simulink model "ASW_PhVltgGen"  (R2023a)
settings: configuration reference "cfg_FastTaskCodeGeneration_v01" (kept outside this file)
undefined symbols (not defined in the file): Cdbl_tiMedTaskSmpTi
settings Model: DataDictionary=dd_foc_dictionary.sldd  EnableAccessToBaseWorkspace=off  Creator=WFYXQ  LastModifiedBy=xiaoqiang.yuan
settings ConfigSetRef: SourceName=cfg_FastTaskCodeGeneration_v01

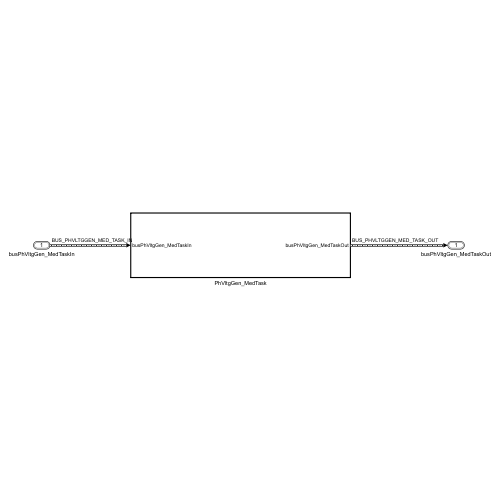
[thumbnail: Simulink's stored preview of the top-level diagram]
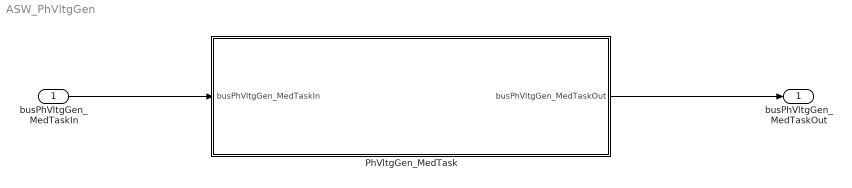
== system ASW_PhVltgGen ==
  busPhVltgGen_MedTaskIn : Inport  OutDataTypeStr=Bus: BUS_PHVLTGGEN_MED_TASK_IN  SampleTime=round(double(Cdbl_tiMedTaskSmpTi),6)  BusOutputAsStruct=on
  PhVltgGen_MedTask : Subsystem  TreatAsAtomicUnit=on  RTWFcnName=PhVltgGen_MedTask
      settings: RTWSystemCode=Nonreusable function  RTWFcnNameOpts=User specified
  busPhVltgGen_MedTaskOut : Outport  OutDataTypeStr=Bus: BUS_PHVLTGGEN_MED_TASK_OUT  SampleTime=round(double(Cdbl_tiMedTaskSmpTi),6)
  wires:
  busPhVltgGen_MedTaskIn/1 -> PhVltgGen_MedTask/1(busPhVltgGen_MedTaskIn)
  PhVltgGen_MedTask/1(busPhVltgGen_MedTaskOut) -> busPhVltgGen_MedTaskOut/1

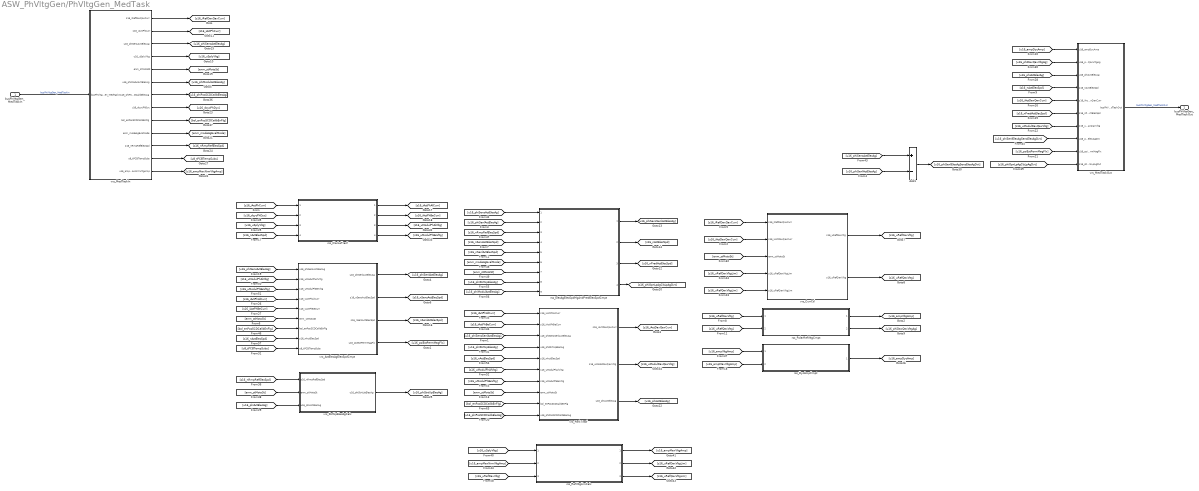
== system ASW_PhVltgGen/PhVltgGen_MedTask ==
  busPhVltgGen_MedTaskIn : Inport
  Add1 : Sum  InitFcn=|  Inputs=+-  OutDataTypeStr=Inherit: Same as first input
      | Simulink.suppressDiagnostic(gcb,...
      | 'SimulinkFixedPoint:util:Overflowoccurred');
  rss_ClarkeTrasf : Subsystem  ReferencedSubsystem=rss_ClarkeTrasf
  rss_DycAmpCmpt : Subsystem  ReferencedSubsystem=rss_DycAmpCmpt
  rss_ElecAgElecSpdMgAndPredElecSpdCmpt : Subsystem  VariantControl=Choice  ReferencedSubsystem=rss_ElecAgElecSpdMgAndPredElecSpdCmpt
  rss_PolarRefVltgCmpt : Subsystem  ReferencedSubsystem=rss_PolarRefVltgCmpt
  rss_RefVltgLimCalc : Subsystem  ReferencedSubsystem=rss_RefVltgLimCalc
  vrs_ActElecAgElecSpdCmpt : Subsystem  Variant=on  VariantControlMode=label  VariantControl=Choice  LabelModeActiveChoice=cstHybrCtrlLbl
  vrs_CurrCtl : Subsystem  Variant=on  VariantControlMode=label  VariantControl=Choice  LabelModeActiveChoice=cstSensCtrlLbl
  vrs_MedTaskIn : Subsystem  Variant=on  VariantControlMode=label  VariantControl=Choice  LabelModeActiveChoice=cstHybrCtrlLbl
  vrs_MedTaskOut : Subsystem  Variant=on  VariantControlMode=label  VariantControl=Choice  LabelModeActiveChoice=cstHybrCtrlLbl
  vrs_ParkTrasf : Subsystem  Variant=on  VariantControlMode=label  VariantControl=cstSensCtrlLbl  LabelModeActiveChoice=cstHybrCtrlLbl
  vrs_StrtUpElecAgCalc : Subsystem  Variant=on  VariantControlMode=label  LabelModeActiveChoice=cstSenlCtrlLbl
  busPhVltgGen_MedTaskOut : Outport
  wires:
  [s16_uModulPhBeVltg] -> vrs_ActElecAgElecSpdCmpt/3(s16_uModulPhBeVltg)
  vrs_MedTaskIn/1(s16_iRefDaxQaxCurr) -> [s16_iRefDaxQaxCurr]
  vrs_MedTaskOut/1(busPhVltgGen_MedTaskOut) -> busPhVltgGen_MedTaskOut/1  "busPhVltgGen_MedTaskOut"
  [u16_phiSensActElecAg] -> vrs_ActElecAgElecSpdCmpt/1(u16_phiSensActElecAg)
  [s16_iActPhCurr] -> rss_ClarkeTrasf/1
  vrs_MedTaskIn/4(u16_uSplyVltg) -> [u16_uSplyVltg]
  [s16_iActDaxQaxCurr] -> vrs_CurrCtl/2(s16_iActDaxQaxCurr)
  [u16_uSplyVltg] -> rss_ClarkeTrasf/3
  vrs_CurrCtl/2(s16_uRefQaxVltg) -> [s16_uRefQaxVltg]
  rss_ClarkeTrasf/1 -> [s16_iActPhAlCurr]
  [s16_uModulDaxQaxVltg] -> vrs_MedTaskOut/7(s16_uModulDaxQaxVltg)
  rss_PolarRefVltgCmpt/1 -> [u16_ampVltgAmp]
  rss_ClarkeTrasf/2 -> [s16_iActPhBeCurr]
  rss_DycAmpCmpt/1 -> [u16_ampDycAmp]
  [u16_ampVltgAmp] -> rss_DycAmpCmpt/1
  [u16_ampMaxVltgAmp] -> rss_DycAmpCmpt/2
  [s16_iActPhAlCurr] -> vrs_ActElecAgElecSpdCmpt/4(s16_iActPhAlCurr)
  [s16_iActPhBeCurr] -> vrs_ActElecAgElecSpdCmpt/5(s16_iActPhBeCurr)
  rss_ClarkeTrasf/3 -> [s16_uModulPhAlVltg]
  busPhVltgGen_MedTaskIn/1 -> vrs_MedTaskIn/1(busPhVltgGen_MedTaskIn)  "busPhVltgGen_MedTaskIn"
  vrs_MedTaskIn/6(u16_phiModulActElecAg) -> [u16_phiModulActElecAg]
  [u16_ampDycAmp] -> vrs_MedTaskOut/1(u16_ampDycAmp)
  rss_ClarkeTrasf/4 -> [s16_uModulPhBeVltg]
  vrs_MedTaskIn/3(u16_phiSensActElecAg) -> [u16_phiSensActElecAg]
  vrs_MedTaskIn/10(enm_modeAgEvalMode) -> [enm_modeAgEvalMode]
  [s16_iRefDaxQaxCurr] -> vrs_CurrCtl/1(s16_iRefDaxQaxCurr)
  [s16_uModulPhAlVltg] -> vrs_ActElecAgElecSpdCmpt/2(s16_uModulPhAlVltg)
  [u16_dcycPhDyc] -> rss_ClarkeTrasf/2
  [s16_nActElecSpd] -> vrs_MedTaskOut/4(s16_nActElecSpd)
  rss_PolarRefVltgCmpt/2 -> [u16_phiDaxQaxVltgAg]
  [s16_uRefDaxVltgLim] -> vrs_CurrCtl/4(s16_uRefDaxVltgLim)
  [s16_iActDaxQaxCurr] -> vrs_MedTaskOut/5(s16_iActDaxQaxCurr)
  [u16_phiDaxQaxVltgAg] -> vrs_MedTaskOut/2(u16_phiDaxQaxVltgAg)
  vrs_MedTaskIn/8(u16_dcycPhDyc) -> [u16_dcycPhDyc]
  vrs_MedTaskIn/7(u16_phiPosSCDCalibElecAg) -> [u16_phiPosSCDCalibElecAg]
  vrs_CurrCtl/1(s16_uRefDaxVltg) -> [s16_uRefDaxVltg]
  vrs_MedTaskIn/5(enm_stMotoSt) -> [enm_stMotoSt]
  vrs_MedTaskIn/2(s16_iActPhCurr) -> [s16_iActPhCurr]
  [u16_phiActElecAg] -> vrs_MedTaskOut/3(u16_phiActElecAg)
  [enm_stMotoSt] -> vrs_CurrCtl/3(enm_stMotoSt)
  vrs_MedTaskIn/9(bol_enPosSCDCalibEnFlg) -> [bol_enPosSCDCalibEnFlg]
  [enm_stMotoSt] -> vrs_ActElecAgElecSpdCmpt/6(enm_stMotoSt)
  [s16_uRefDaxVltg] -> rss_PolarRefVltgCmpt/1
  [s16_uRefQaxVltg] -> rss_PolarRefVltgCmpt/2
  [s16_uRefQaxVltgLim] -> vrs_CurrCtl/5(s16_uRefQaxVltgLim)
  Add1/1 -> [u16_phiSenlElecAgSensElecAgDvt]
  [u16_phiSenlElecAgSensElecAgDvt] -> vrs_MedTaskOut/8(u16_phiSenlElecAgSensElecAgDvt)
  [u16_phiSenlActElecAg] -> Add1/2
  [u16_phiSensActElecAg] -> Add1/1
  [enm_stMotoSt] -> vrs_StrtUpElecAgCalc/2(enm_stMotoSt)
  [u16_phiActElecAg] -> vrs_StrtUpElecAgCalc/3(u16_phiActElecAg)
  [s16_nRmpRefElecSpd] -> vrs_StrtUpElecAgCalc/1(s16_nRmpRefElecSpd)
  vrs_MedTaskIn/11(s16_nRmpRefElecSpd) -> [s16_nRmpRefElecSpd]
  vrs_StrtUpElecAgCalc/1(u16_phiStrtUpElecAg) -> [u16_phiStrtUpElecAg]
  [s16_nPredActElecSpd] -> vrs_MedTaskOut/6(s16_nPredActElecSpd)
  vrs_ActElecAgElecSpdCmpt/2(s16_nSensActElecSpd) -> [s16_nSensActElecSpd]
  vrs_ActElecAgElecSpdCmpt/3(s16_nSenlActElecSpd) -> [s16_nSenlActElecSpd]
  [s16_iActPhAlCurr] -> vrs_ParkTrasf/1(s16_iActPhAlCurr)
  [s16_iActPhBeCurr] -> vrs_ParkTrasf/2(s16_iActPhBeCurr)
  [u16_phiSensSenlActElecAg] -> vrs_ParkTrasf/3(u16_phiSensSenlActElecAg)
  [u16_phiStrtUpElecAg] -> vrs_ParkTrasf/4(u16_phiStrtUpElecAg)
  [s16_nActElecSpd] -> vrs_ParkTrasf/5(s16_nActElecSpd)
  [s16_uModulPhAlVltg] -> vrs_ParkTrasf/6(s16_uModulPhAlVltg)
  [s16_uModulPhBeVltg] -> vrs_ParkTrasf/7(s16_uModulPhBeVltg)
  [enm_stMotoSt] -> vrs_ParkTrasf/8(enm_stMotoSt)
  [bol_enPosSCDCalibEnFlg] -> vrs_ParkTrasf/9(bol_enPosSCDCalibEnFlg)
  [u16_phiPosSCDCalibElecAg] -> vrs_ParkTrasf/10(u16_phiPosSCDCalibElecAg)
  vrs_ParkTrasf/1(s16_iActDaxQaxCurr) -> [s16_iActDaxQaxCurr]
  vrs_ParkTrasf/2(s16_uModulDaxQaxVltg) -> [s16_uModulDaxQaxVltg]
  vrs_ParkTrasf/3(u16_phiActElecAg) -> [u16_phiActElecAg]
  vrs_ActElecAgElecSpdCmpt/4(u16_psiEstPermMagFlx) -> [u16_psiEstPermMagFlx]
  [u16_psiEstPermMagFlx] -> vrs_MedTaskOut/9(u16_psiEstPermMagFlx)
  [bol_enPosSCDCalibEnFlg] -> vrs_ActElecAgElecSpdCmpt/7(bol_enPosSCDCalibEnFlg)
  vrs_ActElecAgElecSpdCmpt/1(u16_phiSenlActElecAg) -> [u16_phiSenlActElecAg]
  [u16_phiSensActElecAg] -> rss_ElecAgElecSpdMgAndPredElecSpdCmpt/1
  [u16_phiSenlActElecAg] -> rss_ElecAgElecSpdMgAndPredElecSpdCmpt/2
  [s16_nRmpRefElecSpd] -> rss_ElecAgElecSpdMgAndPredElecSpdCmpt/3
  [s16_nSensActElecSpd] -> rss_ElecAgElecSpdMgAndPredElecSpdCmpt/4
  [s16_nSenlActElecSpd] -> rss_ElecAgElecSpdMgAndPredElecSpdCmpt/5
  [enm_modeAgEvalMode] -> rss_ElecAgElecSpdMgAndPredElecSpdCmpt/6
  [enm_stMotoSt] -> rss_ElecAgElecSpdMgAndPredElecSpdCmpt/7
  [u16_phiStrtUpElecAg] -> rss_ElecAgElecSpdMgAndPredElecSpdCmpt/8
  [u16_phiModulActElecAg] -> rss_ElecAgElecSpdMgAndPredElecSpdCmpt/9
  rss_ElecAgElecSpdMgAndPredElecSpdCmpt/1 -> [u16_phiSensSenlActElecAg]
  rss_ElecAgElecSpdMgAndPredElecSpdCmpt/2 -> [s16_nActElecSpd]
  rss_ElecAgElecSpdMgAndPredElecSpdCmpt/3 -> [s16_nPredActElecSpd]
  [s16_nActElecSpd] -> vrs_ActElecAgElecSpdCmpt/8(s16_nActElecSpd)
  [s16_nActElecSpd] -> rss_ClarkeTrasf/4
  [u8_tPCBTempSubs] -> vrs_ActElecAgElecSpdCmpt/9(u8_tPCBTempSubs)
  vrs_MedTaskIn/12(u8_tPCBTempSubs) -> [u8_tPCBTempSubs]
  [s16_uRefDaxVltg] -> rss_RefVltgLimCalc/3
  [u16_ampMaxNrmVltgAmp] -> rss_RefVltgLimCalc/2
  [u16_uSplyVltg] -> rss_RefVltgLimCalc/1
  rss_RefVltgLimCalc/2 -> [s16_uRefDaxVltgLim]
  rss_RefVltgLimCalc/3 -> [s16_uRefQaxVltgLim]
  rss_RefVltgLimCalc/1 -> [u16_ampMaxVltgAmp]
  vrs_MedTaskIn/13(u16_ampMaxNrmVltgAmp) -> [u16_ampMaxNrmVltgAmp]
  rss_ElecAgElecSpdMgAndPredElecSpdCmpt/4 -> [s16_phiOpnLpAgClsLpAgDvt]
  [s16_phiOpnLpAgClsLpAgDvt] -> vrs_MedTaskOut/10(s16_phiOpnLpAgClsLpAgDvt)

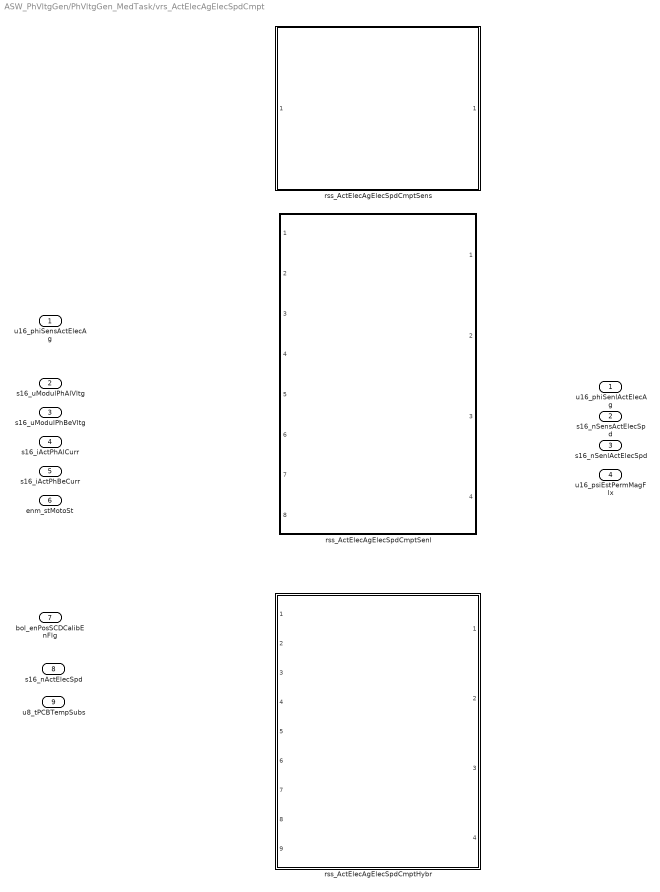
== system ASW_PhVltgGen/PhVltgGen_MedTask/vrs_ActElecAgElecSpdCmpt ==
  u16_phiSensActElecAg : Inport
  s16_uModulPhAlVltg : Inport  Port=2
  s16_uModulPhBeVltg : Inport  Port=3
  s16_iActPhAlCurr : Inport  Port=4
  s16_iActPhBeCurr : Inport  Port=5
  enm_stMotoSt : Inport  Port=6
  bol_enPosSCDCalibEnFlg : Inport  Port=7
  s16_nActElecSpd : Inport  Port=8
  u8_tPCBTempSubs : Inport  Port=9
  rss_ActElecAgElecSpdCmptHybr : Subsystem  VariantControl=cstHybrCtrlLbl  ReferencedSubsystem=rss_ActElecAgElecSpdCmptHybr
  rss_ActElecAgElecSpdCmptSenl : Subsystem  VariantControl=cstSenlCtrlLbl  ReferencedSubsystem=rss_ActElecAgElecSpdCmptSenl
  rss_ActElecAgElecSpdCmptSens : Subsystem  VariantControl=cstSensCtrlLbl  ReferencedSubsystem=rss_ActElecAgElecSpdCmptSens
  u16_phiSenlActElecAg : Outport
  s16_nSensActElecSpd : Outport  Port=2
  s16_nSenlActElecSpd : Outport  Port=3  PortDimensions=1  VectorParamsAs1DForOutWhenUnconnected=off
  u16_psiEstPermMagFlx : Outport  Port=4  PortDimensions=1  VectorParamsAs1DForOutWhenUnconnected=off

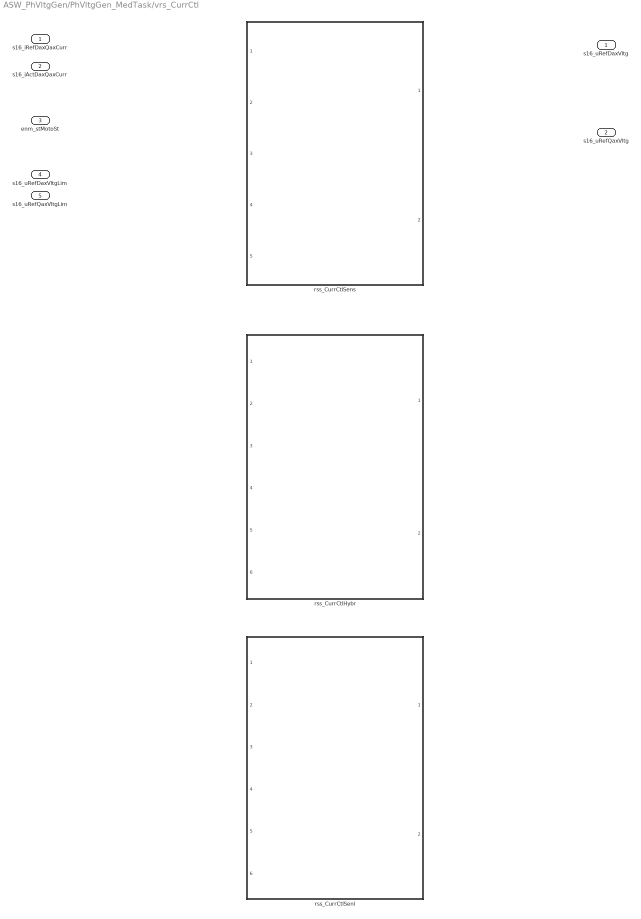
== system ASW_PhVltgGen/PhVltgGen_MedTask/vrs_CurrCtl ==
  s16_iRefDaxQaxCurr : Inport
  s16_iActDaxQaxCurr : Inport  Port=2
  enm_stMotoSt : Inport  Port=3
  s16_uRefDaxVltgLim : Inport  Port=4  OutDataTypeStr=dt_Standardize_s16p15b0
  s16_uRefQaxVltgLim : Inport  Port=5  OutDataTypeStr=dt_Standardize_s16p15b0
  rss_CurrCtlHybr : Subsystem  VariantControl=cstHybrCtrlLbl  ReferencedSubsystem=rss_CurrCtlHybr
  rss_CurrCtlSenl : Subsystem  VariantControl=cstSenlCtrlLbl  ReferencedSubsystem=rss_CurrCtlSenl
  rss_CurrCtlSens : Subsystem  VariantControl=cstSensCtrlLbl  ReferencedSubsystem=rss_CurrCtlSens
  s16_uRefDaxVltg : Outport
  s16_uRefQaxVltg : Outport  Port=2

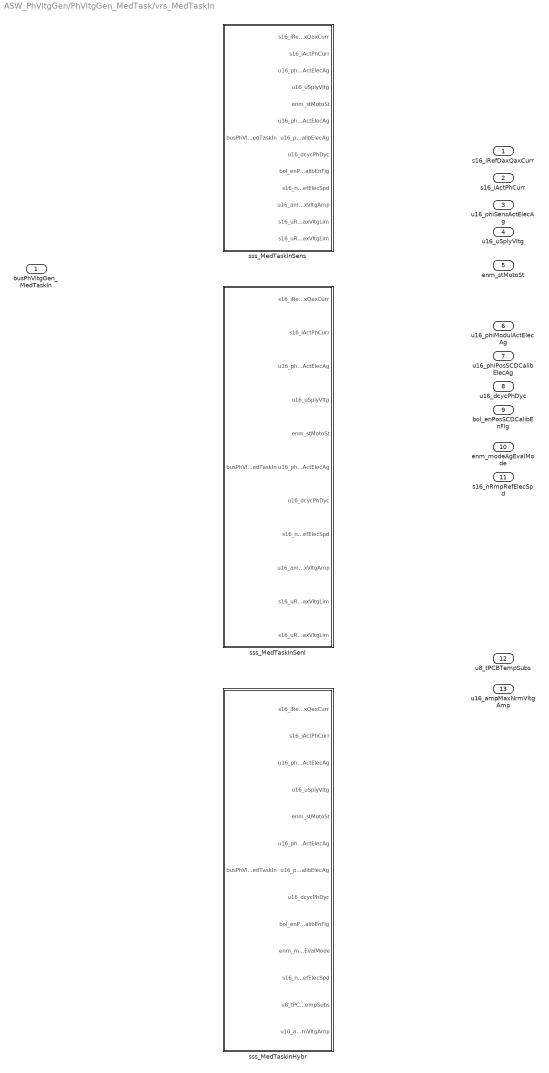
== system ASW_PhVltgGen/PhVltgGen_MedTask/vrs_MedTaskIn ==
  busPhVltgGen_MedTaskIn : Inport
  sss_MedTaskInHybr : Subsystem  VariantControl=cstHybrCtrlLbl
  sss_MedTaskInSenl : Subsystem  VariantControl=cstSenlCtrlLbl
  sss_MedTaskInSens : Subsystem  VariantControl=cstSensCtrlLbl
  s16_iRefDaxQaxCurr : Outport
  s16_iActPhCurr : Outport  Port=2
  u16_phiSensActElecAg : Outport  Port=3
  u16_uSplyVltg : Outport  Port=4
  enm_stMotoSt : Outport  Port=5
  u16_phiModulActElecAg : Outport  Port=6
  u16_phiPosSCDCalibElecAg : Outport  Port=7
  u16_dcycPhDyc : Outport  Port=8
  bol_enPosSCDCalibEnFlg : Outport  Port=9
  enm_modeAgEvalMode : Outport  Port=10
  s16_nRmpRefElecSpd : Outport  Port=11
  u8_tPCBTempSubs : Outport  Port=12
  u16_ampMaxNrmVltgAmp : Outport  Port=13

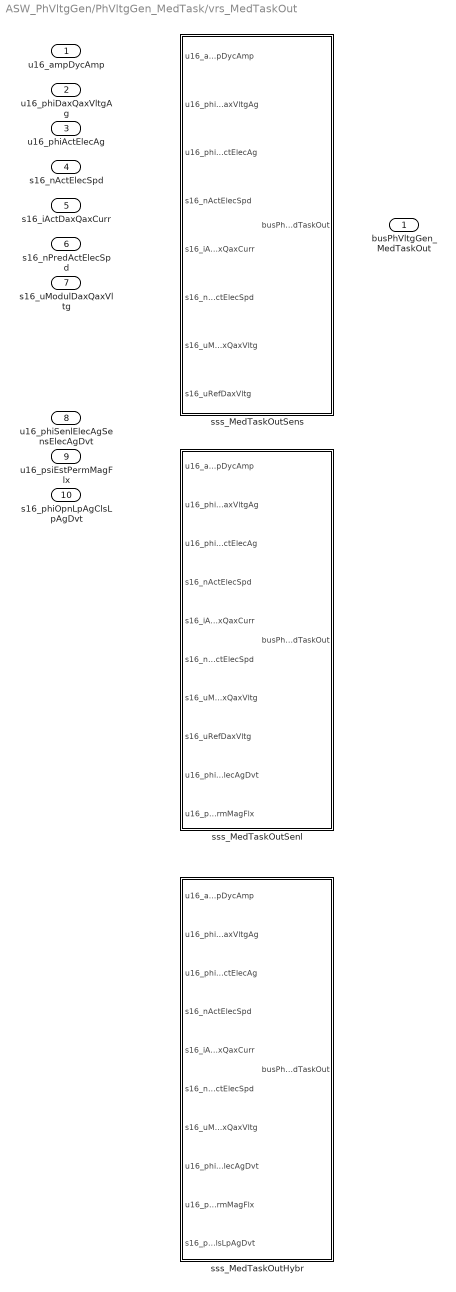
== system ASW_PhVltgGen/PhVltgGen_MedTask/vrs_MedTaskOut ==
  u16_ampDycAmp : Inport
  u16_phiDaxQaxVltgAg : Inport  Port=2
  u16_phiActElecAg : Inport  Port=3
  s16_nActElecSpd : Inport  Port=4
  s16_iActDaxQaxCurr : Inport  Port=5
  s16_nPredActElecSpd : Inport  Port=6
  s16_uModulDaxQaxVltg : Inport  Port=7
  u16_phiSenlElecAgSensElecAgDvt : Inport  Port=8
  u16_psiEstPermMagFlx : Inport  Port=9
  s16_phiOpnLpAgClsLpAgDvt : Inport  Port=10
  sss_MedTaskOutHybr : Subsystem  VariantControl=cstHybrCtrlLbl
  sss_MedTaskOutSenl : Subsystem  VariantControl=cstSenlCtrlLbl
  sss_MedTaskOutSens : Subsystem  VariantControl=cstSensCtrlLbl
  busPhVltgGen_MedTaskOut : Outport

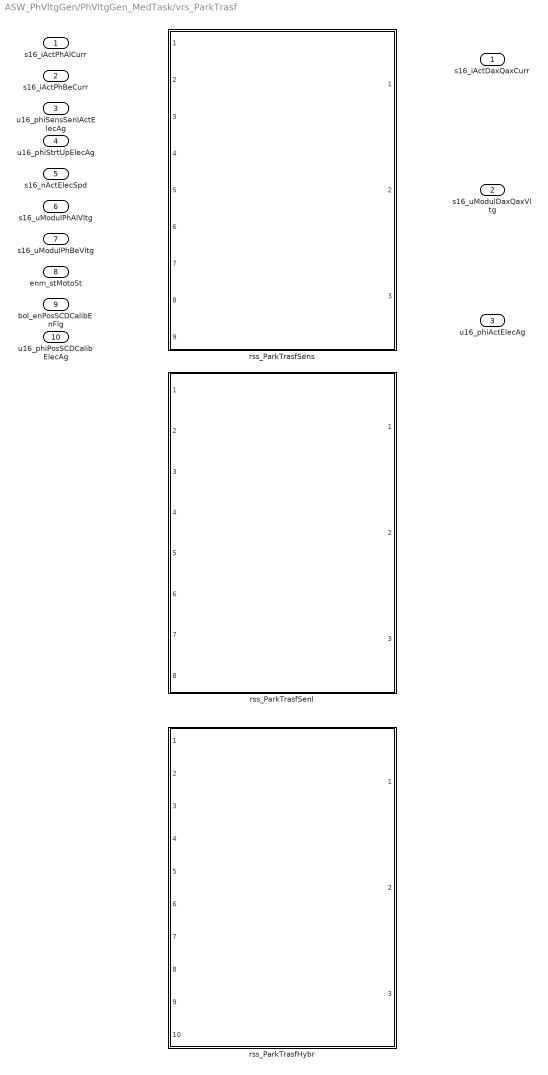
== system ASW_PhVltgGen/PhVltgGen_MedTask/vrs_ParkTrasf ==
  s16_iActPhAlCurr : Inport
  s16_iActPhBeCurr : Inport  Port=2
  u16_phiSensSenlActElecAg : Inport  Port=3
  u16_phiStrtUpElecAg : Inport  Port=4
  s16_nActElecSpd : Inport  Port=5
  s16_uModulPhAlVltg : Inport  Port=6
  s16_uModulPhBeVltg : Inport  Port=7
  enm_stMotoSt : Inport  Port=8
  bol_enPosSCDCalibEnFlg : Inport  Port=9
  u16_phiPosSCDCalibElecAg : Inport  Port=10
  rss_ParkTrasfHybr : Subsystem  InitFcn=|  VariantControl=cstHybrCtrlLbl  ReferencedSubsystem=rss_ParkTrasfHybr
      | Simulink.suppressDiagnostic([gcb,'/Add1'],...
      | 'SimulinkFixedPoint:util:Overflowoccurred');
  rss_ParkTrasfSenl : Subsystem  InitFcn=|  VariantControl=cstSenlCtrlLbl  ReferencedSubsystem=rss_ParkTrasfSenl
      | Simulink.suppressDiagnostic([gcb,'/Add1'],...
      | 'SimulinkFixedPoint:util:Overflowoccurred');
  rss_ParkTrasfSens : Subsystem  VariantControl=cstSensCtrlLbl  ReferencedSubsystem=rss_ParkTrasfSens
  s16_iActDaxQaxCurr : Outport
  s16_uModulDaxQaxVltg : Outport  Port=2
  u16_phiActElecAg : Outport  Port=3

== system ASW_PhVltgGen/PhVltgGen_MedTask/vrs_StrtUpElecAgCalc ==
  note: 1) Add Subsystem or Model blocks as valid variant choices.
      | 2) You cannot connect blocks at this level. At simulation, connectivity is automatically
      | determined, based on the active variant and port name matching.
  s16_nRmpRefElecSpd : Inport
  enm_stMotoSt : Inport  Port=2  PortDimensions=1
  u16_phiActElecAg : Inport  Port=3  PortDimensions=1
  rss_StrtUpElecAgCalcNeed : Subsystem  VariantControl=cstSenlCtrlLbl  ReferencedSubsystem=rss_StrtUpElecAgCalcNeed
  sss_StrtUpElecAgCalcNoNeed : Subsystem  VariantControl=cstSensCtrlLbl
  u16_phiStrtUpElecAg : Outport

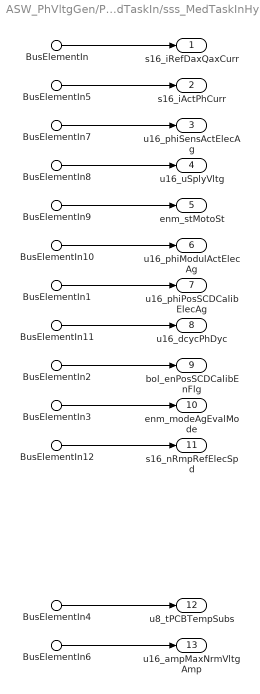
== system ASW_PhVltgGen/PhVltgGen_MedTask/vrs_MedTaskIn/sss_MedTaskInHybr ==
  BusElementIn : Inport  PortName=busPhVltgGen_MedTaskIn  Element=s16_iRefDaxQaxCurr
  BusElementIn5 : Inport  PortName=busPhVltgGen_MedTaskIn  Element=s16_iActPhCurr
  BusElementIn7 : Inport  PortName=busPhVltgGen_MedTaskIn  Element=u16_phiSensActElecAg
  BusElementIn8 : Inport  PortName=busPhVltgGen_MedTaskIn  Element=u16_uSplyVltg
  BusElementIn9 : Inport  PortName=busPhVltgGen_MedTaskIn  Element=enm_stMotoSt
  BusElementIn10 : Inport  PortName=busPhVltgGen_MedTaskIn  Element=u16_phiModulActElecAg
  BusElementIn11 : Inport  PortName=busPhVltgGen_MedTaskIn  Element=u16_dcycPhDyc
  BusElementIn12 : Inport  PortName=busPhVltgGen_MedTaskIn  Element=s16_nRmpRefElecSpd
  BusElementIn1 : Inport  PortName=busPhVltgGen_MedTaskIn  Element=u16_phiPosSCDCalibElecAg
  BusElementIn2 : Inport  PortName=busPhVltgGen_MedTaskIn  Element=bol_enPosSCDCalibEnFlg
  BusElementIn3 : Inport  PortName=busPhVltgGen_MedTaskIn  Element=enm_modeAgEvalMode
  BusElementIn4 : Inport  PortName=busPhVltgGen_MedTaskIn  Element=u8_tPCBTempSubs
  BusElementIn6 : Inport  PortName=busPhVltgGen_MedTaskIn  Element=u16_ampMaxNrmVltgAmp
  s16_iRefDaxQaxCurr : Outport
  s16_iActPhCurr : Outport  Port=2
  u16_phiSensActElecAg : Outport  Port=3  OutDataTypeStr=dt_RadAng_u16r15b0
  u16_uSplyVltg : Outport  Port=4
  enm_stMotoSt : Outport  Port=5
  u16_phiModulActElecAg : Outport  Port=6
  u16_phiPosSCDCalibElecAg : Outport  Port=7
  u16_dcycPhDyc : Outport  Port=8
  bol_enPosSCDCalibEnFlg : Outport  Port=9
  enm_modeAgEvalMode : Outport  Port=10
  s16_nRmpRefElecSpd : Outport  Port=11
  u8_tPCBTempSubs : Outport  Port=12
  u16_ampMaxNrmVltgAmp : Outport  Port=13
  wires:
  BusElementIn12/1 -> s16_nRmpRefElecSpd/1
  BusElementIn8/1 -> u16_uSplyVltg/1
  BusElementIn/1 -> s16_iRefDaxQaxCurr/1
  BusElementIn7/1 -> u16_phiSensActElecAg/1
  BusElementIn9/1 -> enm_stMotoSt/1
  BusElementIn11/1 -> u16_dcycPhDyc/1
  BusElementIn10/1 -> u16_phiModulActElecAg/1
  BusElementIn5/1 -> s16_iActPhCurr/1
  BusElementIn1/1 -> u16_phiPosSCDCalibElecAg/1
  BusElementIn2/1 -> bol_enPosSCDCalibEnFlg/1
  BusElementIn3/1 -> enm_modeAgEvalMode/1
  BusElementIn4/1 -> u8_tPCBTempSubs/1
  BusElementIn6/1 -> u16_ampMaxNrmVltgAmp/1

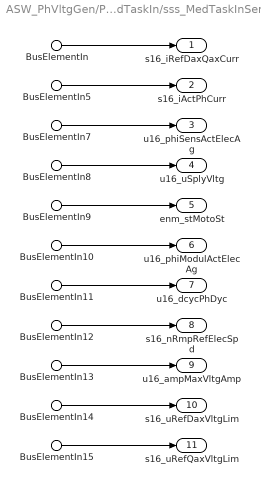
== system ASW_PhVltgGen/PhVltgGen_MedTask/vrs_MedTaskIn/sss_MedTaskInSenl ==
  BusElementIn : Inport  PortName=busPhVltgGen_MedTaskIn  Element=s16_iRefDaxQaxCurr
  BusElementIn5 : Inport  PortName=busPhVltgGen_MedTaskIn  Element=s16_iActPhCurr
  BusElementIn7 : Inport  PortName=busPhVltgGen_MedTaskIn  Element=u16_phiSensActElecAg
  BusElementIn8 : Inport  PortName=busPhVltgGen_MedTaskIn  Element=u16_uSplyVltg
  BusElementIn9 : Inport  PortName=busPhVltgGen_MedTaskIn  Element=enm_stMotoSt
  BusElementIn10 : Inport  PortName=busPhVltgGen_MedTaskIn  Element=u16_phiModulActElecAg
  BusElementIn11 : Inport  PortName=busPhVltgGen_MedTaskIn  Element=u16_dcycPhDyc
  BusElementIn12 : Inport  PortName=busPhVltgGen_MedTaskIn  Element=s16_nRmpRefElecSpd
  BusElementIn13 : Inport  PortName=busPhVltgGen_MedTaskIn  Element=u16_ampMaxVltgAmp
  BusElementIn14 : Inport  PortName=busPhVltgGen_MedTaskIn  Element=s16_uRefDaxVltgLim
  BusElementIn15 : Inport  PortName=busPhVltgGen_MedTaskIn  Element=s16_uRefQaxVltgLim
  s16_iRefDaxQaxCurr : Outport
  s16_iActPhCurr : Outport  Port=2
  u16_phiSensActElecAg : Outport  Port=3  OutDataTypeStr=dt_RadAng_u16r15b0
  u16_uSplyVltg : Outport  Port=4
  enm_stMotoSt : Outport  Port=5
  u16_phiModulActElecAg : Outport  Port=6
  u16_dcycPhDyc : Outport  Port=7
  s16_nRmpRefElecSpd : Outport  Port=8
  u16_ampMaxVltgAmp : Outport  Port=9
  s16_uRefDaxVltgLim : Outport  Port=10
  s16_uRefQaxVltgLim : Outport  Port=11
  wires:
  BusElementIn/1 -> s16_iRefDaxQaxCurr/1
  BusElementIn5/1 -> s16_iActPhCurr/1
  BusElementIn8/1 -> u16_uSplyVltg/1
  BusElementIn9/1 -> enm_stMotoSt/1
  BusElementIn10/1 -> u16_phiModulActElecAg/1
  BusElementIn11/1 -> u16_dcycPhDyc/1
  BusElementIn12/1 -> s16_nRmpRefElecSpd/1
  BusElementIn15/1 -> s16_uRefQaxVltgLim/1
  BusElementIn7/1 -> u16_phiSensActElecAg/1
  BusElementIn13/1 -> u16_ampMaxVltgAmp/1
  BusElementIn14/1 -> s16_uRefDaxVltgLim/1

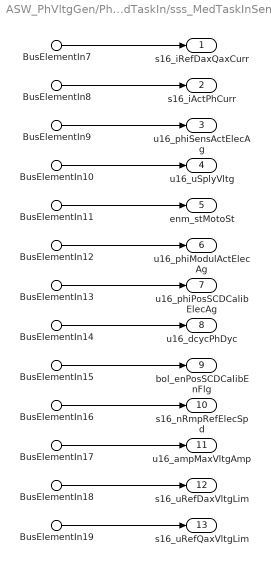
== system ASW_PhVltgGen/PhVltgGen_MedTask/vrs_MedTaskIn/sss_MedTaskInSens ==
  BusElementIn7 : Inport  PortName=busPhVltgGen_MedTaskIn  Element=s16_iRefDaxQaxCurr
  BusElementIn8 : Inport  PortName=busPhVltgGen_MedTaskIn  Element=s16_iActPhCurr
  BusElementIn9 : Inport  PortName=busPhVltgGen_MedTaskIn  Element=u16_phiSensActElecAg
  BusElementIn10 : Inport  PortName=busPhVltgGen_MedTaskIn  Element=u16_uSplyVltg
  BusElementIn11 : Inport  PortName=busPhVltgGen_MedTaskIn  Element=enm_stMotoSt
  BusElementIn12 : Inport  PortName=busPhVltgGen_MedTaskIn  Element=u16_phiModulActElecAg
  BusElementIn13 : Inport  PortName=busPhVltgGen_MedTaskIn  Element=u16_phiPosSCDCalibElecAg
  BusElementIn14 : Inport  PortName=busPhVltgGen_MedTaskIn  Element=u16_dcycPhDyc
  BusElementIn15 : Inport  PortName=busPhVltgGen_MedTaskIn  Element=bol_enPosSCDCalibEnFlg
  BusElementIn16 : Inport  PortName=busPhVltgGen_MedTaskIn  Element=s16_nRmpRefElecSpd
  BusElementIn17 : Inport  PortName=busPhVltgGen_MedTaskIn  Element=u16_ampMaxVltgAmp
  BusElementIn18 : Inport  PortName=busPhVltgGen_MedTaskIn  Element=s16_uRefDaxVltgLim
  BusElementIn19 : Inport  PortName=busPhVltgGen_MedTaskIn  Element=s16_uRefQaxVltgLim
  s16_iRefDaxQaxCurr : Outport
  s16_iActPhCurr : Outport  Port=2
  u16_phiSensActElecAg : Outport  Port=3
  u16_uSplyVltg : Outport  Port=4
  enm_stMotoSt : Outport  Port=5
  u16_phiModulActElecAg : Outport  Port=6
  u16_phiPosSCDCalibElecAg : Outport  Port=7
  u16_dcycPhDyc : Outport  Port=8
  bol_enPosSCDCalibEnFlg : Outport  Port=9
  s16_nRmpRefElecSpd : Outport  Port=10
  u16_ampMaxVltgAmp : Outport  Port=11
  s16_uRefDaxVltgLim : Outport  Port=12
  s16_uRefQaxVltgLim : Outport  Port=13
  wires:
  BusElementIn7/1 -> s16_iRefDaxQaxCurr/1
  BusElementIn8/1 -> s16_iActPhCurr/1
  BusElementIn9/1 -> u16_phiSensActElecAg/1
  BusElementIn10/1 -> u16_uSplyVltg/1
  BusElementIn11/1 -> enm_stMotoSt/1
  BusElementIn12/1 -> u16_phiModulActElecAg/1
  BusElementIn13/1 -> u16_phiPosSCDCalibElecAg/1
  BusElementIn14/1 -> u16_dcycPhDyc/1
  BusElementIn15/1 -> bol_enPosSCDCalibEnFlg/1
  BusElementIn16/1 -> s16_nRmpRefElecSpd/1
  BusElementIn17/1 -> u16_ampMaxVltgAmp/1
  BusElementIn18/1 -> s16_uRefDaxVltgLim/1
  BusElementIn19/1 -> s16_uRefQaxVltgLim/1

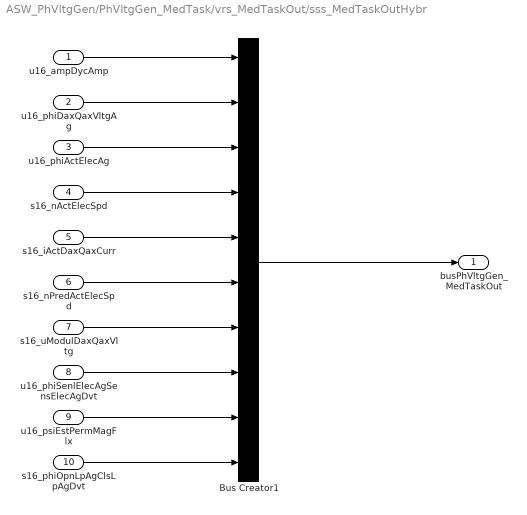
== system ASW_PhVltgGen/PhVltgGen_MedTask/vrs_MedTaskOut/sss_MedTaskOutHybr ==
  u16_ampDycAmp : Inport
  u16_phiDaxQaxVltgAg : Inport  Port=2
  u16_phiActElecAg : Inport  Port=3
  s16_nActElecSpd : Inport  Port=4
  s16_iActDaxQaxCurr : Inport  Port=5
  s16_nPredActElecSpd : Inport  Port=6
  s16_uModulDaxQaxVltg : Inport  Port=7
  u16_phiSenlElecAgSensElecAgDvt : Inport  Port=8
  u16_psiEstPermMagFlx : Inport  Port=9
  s16_phiOpnLpAgClsLpAgDvt : Inport  Port=10
  Bus Creator1 : BusCreator  Inputs=10  OutDataTypeStr=Bus: BUS_PHVLTGGEN_MED_TASK_OUT  NonVirtualBus=on
      settings: InheritFromInputs=off
  busPhVltgGen_MedTaskOut : Outport
  wires:
  u16_psiEstPermMagFlx/1 -> Bus Creator1/9
  Bus Creator1/1 -> busPhVltgGen_MedTaskOut/1
  u16_ampDycAmp/1 -> Bus Creator1/1
  s16_nPredActElecSpd/1 -> Bus Creator1/6
  u16_phiActElecAg/1 -> Bus Creator1/3
  u16_phiDaxQaxVltgAg/1 -> Bus Creator1/2
  s16_nActElecSpd/1 -> Bus Creator1/4
  s16_uModulDaxQaxVltg/1 -> Bus Creator1/7
  s16_iActDaxQaxCurr/1 -> Bus Creator1/5
  u16_phiSenlElecAgSensElecAgDvt/1 -> Bus Creator1/8
  s16_phiOpnLpAgClsLpAgDvt/1 -> Bus Creator1/10

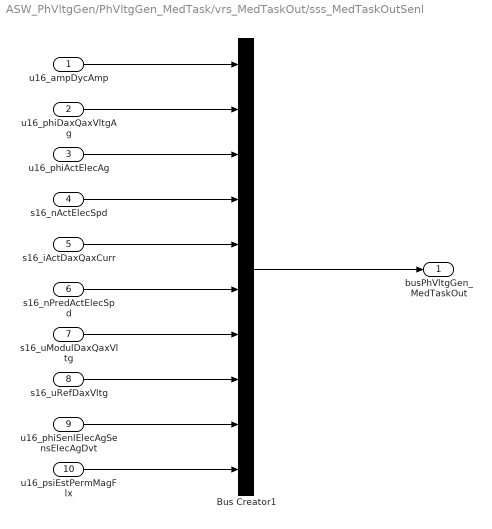
== system ASW_PhVltgGen/PhVltgGen_MedTask/vrs_MedTaskOut/sss_MedTaskOutSenl ==
  u16_ampDycAmp : Inport
  u16_phiDaxQaxVltgAg : Inport  Port=2
  u16_phiActElecAg : Inport  Port=3
  s16_nActElecSpd : Inport  Port=4
  s16_iActDaxQaxCurr : Inport  Port=5
  s16_nPredActElecSpd : Inport  Port=6
  s16_uModulDaxQaxVltg : Inport  Port=7
  s16_uRefDaxVltg : Inport  Port=8
  u16_phiSenlElecAgSensElecAgDvt : Inport  Port=9
  u16_psiEstPermMagFlx : Inport  Port=10
  Bus Creator1 : BusCreator  Inputs=10  OutDataTypeStr=Bus: BUS_PHVLTGGEN_MED_TASK_OUT  NonVirtualBus=on
      settings: InheritFromInputs=off
  busPhVltgGen_MedTaskOut : Outport
  wires:
  s16_iActDaxQaxCurr/1 -> Bus Creator1/5
  s16_nActElecSpd/1 -> Bus Creator1/4
  u16_ampDycAmp/1 -> Bus Creator1/1
  u16_phiDaxQaxVltgAg/1 -> Bus Creator1/2
  s16_nPredActElecSpd/1 -> Bus Creator1/6
  u16_phiActElecAg/1 -> Bus Creator1/3
  s16_uModulDaxQaxVltg/1 -> Bus Creator1/7
  s16_uRefDaxVltg/1 -> Bus Creator1/8
  u16_phiSenlElecAgSensElecAgDvt/1 -> Bus Creator1/9
  Bus Creator1/1 -> busPhVltgGen_MedTaskOut/1
  u16_psiEstPermMagFlx/1 -> Bus Creator1/10

== system ASW_PhVltgGen/PhVltgGen_MedTask/vrs_MedTaskOut/sss_MedTaskOutSens ==
  u16_ampDycAmp : Inport
  u16_phiDaxQaxVltgAg : Inport  Port=2
  u16_phiActElecAg : Inport  Port=3
  s16_nActElecSpd : Inport  Port=4
  s16_iActDaxQaxCurr : Inport  Port=5
  s16_nPredActElecSpd : Inport  Port=6
  s16_uModulDaxQaxVltg : Inport  Port=7
  s16_uRefDaxVltg : Inport  Port=8  OutDataTypeStr=dt_Standardize_s16p15b0
  Bus Creator1 : BusCreator  Inputs=8  OutDataTypeStr=Bus: BUS_PHVLTGGEN_MED_TASK_OUT  NonVirtualBus=on
      settings: InheritFromInputs=off
  busPhVltgGen_MedTaskOut : Outport
  wires:
  s16_iActDaxQaxCurr/1 -> Bus Creator1/5
  s16_nActElecSpd/1 -> Bus Creator1/4
  u16_ampDycAmp/1 -> Bus Creator1/1
  u16_phiDaxQaxVltgAg/1 -> Bus Creator1/2
  s16_nPredActElecSpd/1 -> Bus Creator1/6
  u16_phiActElecAg/1 -> Bus Creator1/3
  s16_uModulDaxQaxVltg/1 -> Bus Creator1/7
  s16_uRefDaxVltg/1 -> Bus Creator1/8
  Bus Creator1/1 -> busPhVltgGen_MedTaskOut/1

== system ASW_PhVltgGen/PhVltgGen_MedTask/vrs_StrtUpElecAgCalc/sss_StrtUpElecAgCalcNoNeed ==
